simulink model "F16ASYM_Controlled_AoA"  (R2012b)
settings: Solver=ode3  SolverMode=SingleTasking  StartTime=0.0  StopTime=inf  FixedStep=T_sim  RelTol=1e-3
InitFcn:
  | load('NN_c_weights_Last_stable.mat')
values from neighbouring files (symbols this model uses):
  K_b_AoA = params(3)    [Cost_function.m]
  K_b_q = params(4)    [Cost_function.m]
  learning = 20    [Scheduling_desing.m]
  Model_used_flag = 1    [Scheduling_desing.m]
  reg_param = 0.5    [Scheduling_desing.m]
  T_sim = 0.02    [Scheduling_desing.m]
  tau_AoA = params(1)    [Cost_function.m]
  tau_q = params(2)    [Cost_function.m]
  Theta_1_roll_last = [0.00183613313267 0.00115998993235 0.0006676025148 0.00194921904952 0.00134963559861 0.00034352059664 0.000447169388141 0.00146749660935 0.00110199952389 7.77922383894e-05 0.00109492833348 0.00192687590535 ... (360 elements, 30x12)]    [NN_i_weights_LAST_STABLE.mat]
  Theta_2_roll_last = [0.000469743069697 0.000355923851088 0.00180035760697 0.00191855117771 0.00118851504447 0.0013331642065 0.0013164316578 0.000643981263341 0.00176817665434 0.000113802099363 0.000426534542462 0.00113815782354 ... (620 elements, 20x31)]    [NN_i_weights_LAST_STABLE.mat]
  Theta_3_roll_last = [9.62071520568e-05 -0.000389870886846 2.08260845013e-05 0.000140787743673 -0.000917525755397 -0.0014324207578 -0.00154701573815 -0.00131544476264 -0.00101205584381 5.06515794689e-05 -0.00111443483676 -0.00143957416141 ... (21 elements, 1x21)]    [NN_i_weights_LAST_STABLE.mat]
  V_long_lastA_w_z = [0.352826086601 -0.253633004548 -0.642535042878 0.237749930435 -0.618390629538 0.858074761295 0.268211230628 -0.448715080196 -0.0406384631192 0.401147605577 0.60598427709 0.0500551915851 ... (300 elements, 30x10)]    [NN_i_weights_LAST_STABLE.mat]
  V_long_lastAoA = [0.0774300162379 0.0911421319631 0.0352371192557 0.0542170286952 0.0651171200844 0.0177112012707 0.0982957728448 0.000259994642558 0.0194724569123 0.0466321328252 0.0556687953852 0.0252668067142 ... (300 elements, 30x10)]    [NN_i_weights_LAST_STABLE.mat]
  V_roll_last = [0.0540918675943 0.0557493347212 0.0839792276608 0.0460576391794 0.0671229058124 0.100220403067 0.0722493281881 0.0648875457457 0.00447599349201 0.0607299103823 0.0488037966361 0.0176785979393 ... (360 elements, 30x12)]    [NN_i_weights_LAST_STABLE.mat]
  V_yaw_last = [0.0965149149679 0.00833616709545 0.0365734360076 0.0523944217566 0.00790252078455 0.0700053845887 0.0345164868709 0.0111568465295 0.094060639546 0.0205483560006 0.000798047494256 0.0862769385758 ... (360 elements, 30x12)]    [NN_i_weights_LAST_STABLE.mat]
  velocity = M_eval_sche(I,J)*a    [Scheduling_desing.m]
  W_long_lastA_w_z = [-0.0522913429974 0.00385484301394 -0.00465489482472 -0.0139416219936 0.00295196421483 -0.013027768541 0.00585545058915 0.00278802233571 -0.00906272782329 -0.000396112031465 0.00405849743321 0.00509668457818 ... (31 elements, 1x31)]    [NN_i_weights_LAST_STABLE.mat]
  W_long_lastAoA = [-0.0192589013922 0.00873109909713 0.00432649597332 0.0420946902441 0.0293366820194 0.0351497798191 0.0234952374236 0.0360841187718 0.0112233388211 0.030147202199 0.0369533138617 0.00218839076415 ... (31 elements, 1x31)]    [NN_i_weights_LAST_STABLE.mat]
  W_roll_last = [-0.0006515532842 0.000535485585715 0.000550946920743 0.000806030945453 0.00045976209382 0.00065557954304 0.000945902185602 0.00070191398535 0.000635215543728 4.66501377412e-05 0.000597079583757 0.000485790566765 ... (31 elements, 1x31)]    [NN_i_weights_LAST_STABLE.mat]
  W_yaw_last = [-4.34263633305e-05 8.83823048922e-05 1.65575463724e-05 3.60293102233e-05 5.19752447623e-05 7.06399280852e-06 7.02425975821e-05 3.62680255076e-05 1.29996379937e-05 8.05072914397e-05 2.39941870661e-05 2.52427840574e-06 ... (31 elements, 1x31)]    [NN_i_weights_LAST_STABLE.mat]
undefined symbols (not defined in the file or in its folder): a1, alpha_map_eval, B, beta_map_eval, C_L_0, DiscIntNeverNeededParam, fi_flag_Simulink, G_eval, H_sq, H_sq_autotrim, k_B, m_B, M_sq, M_sq_autotrim, sigbuilder_block, Stall_curve, trim_control, trim_state, trim_throttle, V_Comp_A_w_z_last, V_Comp_last, V_roll_lastMOD, W_Comp_A_w_z_last, W_Comp_last, W_roll_lastMOD
libraries: Adaptive_FaultTolerantControl x43, dspsigops x29, F16_Actuator_Library x14, simulink x8, aerolibatmos2 x7, dsparch4 x6, simulink_extras x5, aerolibtransform2 x5, qcatlib x4, dspmtrx3 x3, dspvision x2, dspsnks4 x2
(part 6 of 11)

== system F16ASYM_Controlled_AoA/Primary Controller/P controller + adaptive Crossed NN/Lat_dir Dyn Inversion: beta_dot->r_c ==
  beta_dot_c : Inport
  All_meas : Inport  Port=2
  A_w_y : Selector  InputPortWidth=3  IndexOptions=Index vector (dialog)  Indices=2  OutputSizes=1
  Bus Selector : BusSelector  OutputSignals=signal1.AoA meas (rad),signal1.omega_b meas (rad/s),signal1.V_TAS (m/s),signal2.A_w_CG
  Divide1 : Product  Inputs=**
  Divide3 : Product  Inputs=**
  Divide4 : Product  Inputs=/*
  Divide5 : Product  Inputs=*/
  Selector : Selector  InputPortWidth=3  IndexOptions=Index vector (dialog)  Indices=1  OutputSizes=1
  Trigonometric Function : Trigonometry  Operator=cos
  Trigonometric Function3 : Trigonometry  Operator=tan
  "q_c " : Sum  Inputs=-++
  r_c : Outport
  wires:
  Selector/1 -> Divide1/2
  Trigonometric Function3/1 -> Divide1/1
  beta_dot_c/1 -> Divide5/1
  Divide5/1 -> "q_c "/1
  Trigonometric Function/1 -> Divide5/2, Divide3/1
  Bus Selector/3 -> Divide3/2  "<V_TAS (m/s)>"
  Divide4/1 -> "q_c "/3
  Bus Selector/4 -> A_w_y/1  "<A_w_CG>"
  All_meas/1 -> Bus Selector/1
  A_w_y/1 -> Divide4/2
  Divide3/1 -> Divide4/1
  Divide1/1 -> "q_c "/2
  Bus Selector/2 -> Selector/1  "<omega_b meas (rad/s)>"
  Bus Selector/1 -> Trigonometric Function3/1, Trigonometric Function/1  "<AoA meas (rad)>"
  "q_c "/1 -> r_c/1

== system F16ASYM_Controlled_AoA/Primary Controller/P controller + adaptive Crossed NN/Long Dyn Inversion: alpha_dot ->q ==
  alpha_dot_c : Inport
  All_meas : Inport  Port=2
  Completed : Subsystem
  Manual Switch : ManualSwitch
  Simplified : Subsystem
  q_c : Outport
  wires:
  Manual Switch/1 -> q_c/1
  Simplified/1(q_c) -> Manual Switch/2
  Completed/1(q_c) -> Manual Switch/1
  All_meas/1 -> Completed/2(All_meas), Simplified/2(All_meas)
  alpha_dot_c/1 -> Completed/1(alpha_dot_c), Simplified/1(alpha_dot_c)

== system F16ASYM_Controlled_AoA/Primary Controller/P controller + adaptive Crossed NN/Longitudinal Controller: AoA or A_w_z ==
  A_w_z des : Inport
  AoA des (rad) : Inport  Port=2
  Anti-windup A_w_z : Inport  Port=3
  Anti-windup AoA : Inport  Port=4
  All meas : Inport  Port=5
  Longitudinal controller in A_w_z : Subsystem  VariantObject=Controller of A_w_z
  Longitudinal controller in AoA : Subsystem  VariantObject=Controller of AoA
  A_chanel vars : Outport
  alpha_chanel vars : Outport  Port=2
  alpha_dot_c : Outport  Port=3

== system F16ASYM_Controlled_AoA/Primary Controller/P controller + adaptive Crossed NN/Sigmoid  ==
  In : Inport
  Display : Display
  Fcn1 : Fcn  Commented=on  Expr=2.0 ./ (1.0 + exp(-u(4)*u(1:3)))-1
  MATLAB Function : MATLAB Function  TreatAsAtomicUnit=on
  a : Constant  Value=a
  Out : Outport
  wires:
  a/1 -> MATLAB Function/2(a)
  In/1 -> MATLAB Function/1(u)
  MATLAB Function/1(y) -> Out/1, Display/1

== system F16ASYM_Controlled_AoA/Primary Controller/P controller + adaptive Crossed NN + AWU+Lim /Body Rates Controller ==
  p_ref : Inport
  q_ref : Inport  Port=2
  r_ref : Inport  Port=3
  All_meas : Inport  Port=4
  Bus Creator : BusCreator
  Bus Creator1 : BusCreator
  Bus Creator2 : BusCreator
  Bus Selector : BusSelector  OutputSignals=signal1.omega_b meas (rad/s)
  Display1 : Display
  Mux : Mux  Inputs=3
  Ref Model and P Controller p : Adaptive_FaultTolerantControl/Ref Model and P Controller  tau=0.1  y_i=trim_state(10)  K_f=1  K_b=7
  Ref Model and P Controller q : Adaptive_FaultTolerantControl/Ref Model and P Controller  tau=0.25  y_i=trim_state(11)  K_f=1  K_b=6
  Ref Model and P Controller r : Adaptive_FaultTolerantControl/Ref Model and P Controller  tau=0.2  y_i=trim_state(12)  K_f=1  K_b=4
  Selector : Selector  InputPortWidth=3  IndexOptions=Index vector (dialog)  Indices=1  OutputSizes=1
  Selector1 : Selector  InputPortWidth=3  IndexOptions=Index vector (dialog)  Indices=2  OutputSizes=1
  Selector2 : Selector  InputPortWidth=3  IndexOptions=Index vector (dialog)  Indices=3  OutputSizes=1
  Sum : Sum  Inputs=+-|
  Sum1 : Sum  Inputs=+-|
  Sum2 : Sum  Inputs=+-|
  q_chanel vars : Outport
  p_chanel vars : Outport  Port=2
  r_chanel vars : Outport  Port=3
  Angular acc des (rad/s^2) : Outport  Port=4
  wires:
  All_meas/1 -> Bus Selector/1
  Bus Selector/1 -> Selector/1, Selector1/1, Selector2/1  "<omega_b meas (rad/s)>"
  p_ref/1 -> Ref Model and P Controller p/1
  Selector/1 -> Ref Model and P Controller p/2
  Ref Model and P Controller p/1 -> Mux/1
  Mux/1 -> Angular acc des (rad/s^2)/1
  q_ref/1 -> Ref Model and P Controller q/1
  Selector1/1 -> Ref Model and P Controller q/2
  r_ref/1 -> Ref Model and P Controller r/1
  Ref Model and P Controller q/1 -> Mux/2
  Ref Model and P Controller r/1 -> Mux/3
  Ref Model and P Controller p/2 -> Bus Creator/1  "p_sf_dot"
  Ref Model and P Controller p/3 -> Sum/1, Bus Creator/2  "p_sf"
  Sum/1 -> Display1/1, Bus Creator/3  "p_err"
  Bus Creator/1 -> p_chanel vars/1
  Bus Creator1/1 -> q_chanel vars/1
  Bus Creator2/1 -> r_chanel vars/1
  Selector2/1 -> Ref Model and P Controller r/2
  Ref Model and P Controller p/4 -> Sum/2
  Ref Model and P Controller p/5 -> Bus Creator/4  "K_b_p"
  Ref Model and P Controller q/2 -> Bus Creator1/1  "q_sf_dot"
  Ref Model and P Controller q/3 -> Sum1/1, Bus Creator1/2  "q_sf"
  Sum1/1 -> Bus Creator1/3  "q_err"
  Ref Model and P Controller q/4 -> Sum1/2
  Ref Model and P Controller q/5 -> Bus Creator1/4  "K_b_q"
  Ref Model and P Controller r/2 -> Bus Creator2/1  "r_sf_dot"
  Ref Model and P Controller r/3 -> Sum2/1, Bus Creator2/2  "r_sf"
  Sum2/1 -> Bus Creator2/3  "r_err"
  Ref Model and P Controller r/4 -> Sum2/2
  Ref Model and P Controller r/5 -> Bus Creator2/4  "K_b_r"

== system F16ASYM_Controlled_AoA/Primary Controller/P controller + adaptive Crossed NN + AWU+Lim /Complete crossed On-line (adaptive) multi-layer NN ==
  v_ad^ prev : Inport
  All_meas : Inport  Port=2
  NN variables : Inport  Port=3
  AWU : Inport  Port=4
  Complete crossed On-line (adaptive) multi-layer NN: A_w_z : Subsystem  VariantObject=NN on A_w_z
  Complete crossed On-line (adaptive) multi-layer NN: AoA : Subsystem  VariantObject=NN on AoA
  v_ad^ : Outport

== system F16ASYM_Controlled_AoA/Primary Controller/P controller + adaptive Crossed NN + AWU+Lim /Lat_dir Dyn Inversion: beta_dot->r_c ==
  beta_dot_c : Inport
  All_meas : Inport  Port=2
  A_w_y : Selector  InputPortWidth=3  IndexOptions=Index vector (dialog)  Indices=2  OutputSizes=1
  Bus Selector : BusSelector  OutputSignals=signal1.AoA meas (rad),signal1.omega_b meas (rad/s),signal1.V_TAS (m/s),signal2.A_w_CG
  Divide1 : Product  Inputs=**
  Divide3 : Product  Inputs=**
  Divide4 : Product  Inputs=/*
  Divide5 : Product  Inputs=*/
  Selector : Selector  InputPortWidth=3  IndexOptions=Index vector (dialog)  Indices=1  OutputSizes=1
  Trigonometric Function : Trigonometry  Operator=cos
  Trigonometric Function3 : Trigonometry  Operator=tan
  "q_c " : Sum  Inputs=-++
  r_c : Outport
  wires:
  "q_c "/1 -> r_c/1
  Bus Selector/1 -> Trigonometric Function/1, Trigonometric Function3/1  "<AoA meas (rad)>"
  Bus Selector/2 -> Selector/1  "<omega_b meas (rad/s)>"
  Divide1/1 -> "q_c "/2
  Divide3/1 -> Divide4/1
  A_w_y/1 -> Divide4/2
  All_meas/1 -> Bus Selector/1
  Bus Selector/4 -> A_w_y/1  "<A_w_CG>"
  Divide4/1 -> "q_c "/3
  Bus Selector/3 -> Divide3/2  "<V_TAS (m/s)>"
  Trigonometric Function/1 -> Divide3/1, Divide5/2
  Divide5/1 -> "q_c "/1
  beta_dot_c/1 -> Divide5/1
  Trigonometric Function3/1 -> Divide1/1
  Selector/1 -> Divide1/2

== system F16ASYM_Controlled_AoA/Primary Controller/P controller + adaptive Crossed NN + AWU+Lim /Long Dyn Inversion: alpha_dot ->q ==
  alpha_dot_c : Inport
  All_meas : Inport  Port=2
  Completed : Subsystem
  Manual Switch : ManualSwitch
  Simplified : Subsystem
  q_c : Outport
  wires:
  alpha_dot_c/1 -> Simplified/1(alpha_dot_c), Completed/1(alpha_dot_c)
  All_meas/1 -> Simplified/2(All_meas), Completed/2(All_meas)
  Completed/1(q_c) -> Manual Switch/1
  Simplified/1(q_c) -> Manual Switch/2
  Manual Switch/1 -> q_c/1

== system F16ASYM_Controlled_AoA/Primary Controller/P controller + adaptive Crossed NN + AWU+Lim /Longitudinal Controller: AoA or A_w_z ==
  A_w_z des : Inport
  AoA des (rad) : Inport  Port=2
  Anti-windup A_w_z : Inport  Port=3
  Anti-windup AoA : Inport  Port=4
  All meas : Inport  Port=5
  Longitudinal controller in A_w_z : Subsystem  VariantObject=Controller of A_w_z
  Longitudinal controller in AoA : Subsystem  VariantObject=Controller of AoA
  A_chanel vars : Outport
  alpha_chanel vars : Outport  Port=2
  alpha_dot_c : Outport  Port=3

== system F16ASYM_Controlled_AoA/Primary Controller/P controller + adaptive Crossed NN + AWU+Lim /Physical limitation ==
  note: Converto to Angular accelerations
  v comm : Inport
  all meas : Inport  Port=2
  Ang Accel : MATLAB Function
  Bus Selector : BusSelector  OutputSignals=signal1.Alt meas (m),signal1.V_TAS (m/s),signal1.AoA meas (rad),signal1.SS meas (rad),signal1.omega_b meas (rad/s),signal1.Throttle_meas
  Bus Selector1 : BusSelector  OutputSignals=signal2.q (Pa),signal1.omega_b meas (rad/s)
  Demux : Demux  Outputs=3
  Display : Display
  Display1 : Display
  Display2 : Display
  Divide : Product  Inputs=**
  Divide1 : Product  Inputs=**
  Gain : Gain  Gain=-1
  Gain1 : Gain
  Mom coefficients that was reached : MATLABFcn  MATLABFcn=Moms_Coeff_estimator  OutputDimensions=3  OutputSignalType=real
  Moments : Subsystem
  Mux : Mux  Inputs=3
  Mux1 : Mux  Inputs=7
  Saturation Dynamic : simulink/Discontinuities/Saturation Dynamic  OutMin=[]  OutMax=[]  OutDataTypeStr=Inherit: Same as second input  OutDataType=fixdt(1, 16)  OutScaling=2^-10  DoSatur=off
  Sign : Signum
  Sign1 : Signum
  max deflections estimator : MATLAB Function  TreatAsAtomicUnit=on
  v limted : Outport
  wires:
  max deflections estimator/1(max_defl) -> Mux1/7
  Mux1/1 -> Mom coefficients that was reached/1
  Bus Selector/5 -> Mux1/5  "<omega_b meas (rad/s)>"
  Bus Selector/1 -> Mux1/1  "<Alt meas (m)>"
  Bus Selector/2 -> Mux1/2  "<V_TAS (m/s)>"
  Bus Selector/3 -> Mux1/3  "<AoA meas (rad)>"
  Bus Selector/4 -> Mux1/4  "<SS meas (rad)>"
  Bus Selector/6 -> Mux1/6  "<Throttle_meas>"
  Ang Accel/2(q_dot) -> Mux/2
  Ang Accel/3(r_dot) -> Mux/3
  Ang Accel/1(p_dot) -> Mux/1
  Bus Selector1/2 -> Ang Accel/4(omega_b)  "<omega_b meas (rad/s)>"
  Moments/3(N) -> Ang Accel/3(N)
  Moments/2(M) -> Ang Accel/2(M)
  Moments/1(L) -> Ang Accel/1(L)
  Bus Selector1/1 -> Moments/4(q)  "<q (Pa)>"
  Demux/3 -> Moments/3(C_N)
  Demux/2 -> Moments/2(C_M)
  Demux/1 -> Moments/1(C_L)
  Mom coefficients that was reached/1 -> Demux/1
  all meas/1 -> Bus Selector/1, Bus Selector1/1
  Mux/1 -> Gain1/1
  v comm/1 -> Saturation Dynamic/2, Display1/1, max deflections estimator/1(v_comm)
  Saturation Dynamic/1 -> Display/1, v limted/1
  Sign/1 -> Divide/1
  Gain1/1 -> Divide/2, Divide1/1, Sign1/1, Display2/1, Sign/1
  Sign1/1 -> Gain/1
  Divide/1 -> Saturation Dynamic/1
  Gain/1 -> Divide1/2
  Divide1/1 -> Saturation Dynamic/3

== system F16ASYM_Controlled_AoA/Primary Controller/P controller + adaptive Crossed NN + AWU+Lim /Sigmoid  ==
  In : Inport
  Display : Display
  Fcn1 : Fcn  Commented=on  Expr=2.0 ./ (1.0 + exp(-u(4)*u(1:3)))-1
  MATLAB Function : MATLAB Function  TreatAsAtomicUnit=on
  a : Constant  Value=a
  Out : Outport
  wires:
  MATLAB Function/1(y) -> Display/1, Out/1
  In/1 -> MATLAB Function/1(u)
  a/1 -> MATLAB Function/2(a)

== system F16ASYM_Controlled_AoA/Primary Controller/P controller + adaptive Isolated NN/Body Rates Controller ==
  p_ref : Inport
  q_ref : Inport  Port=2
  r_ref : Inport  Port=3
  All_meas : Inport  Port=4
  Bus Creator : BusCreator
  Bus Creator1 : BusCreator
  Bus Creator2 : BusCreator
  Bus Selector : BusSelector  OutputSignals=signal1.omega_b meas (rad/s)
  Display1 : Display
  Mux : Mux  Inputs=3
  Ref Model and P Controller p : Adaptive_FaultTolerantControl/Ref Model and P Controller  tau=0.1  y_i=trim_state(10)  K_f=1  K_b=7
  Ref Model and P Controller q : Adaptive_FaultTolerantControl/Ref Model and P Controller  tau=0.25  y_i=trim_state(11)  K_f=1  K_b=8
  Ref Model and P Controller r : Adaptive_FaultTolerantControl/Ref Model and P Controller  tau=0.2  y_i=trim_state(12)  K_f=1  K_b=4
  Selector : Selector  InputPortWidth=3  IndexOptions=Index vector (dialog)  Indices=1  OutputSizes=1
  Selector1 : Selector  InputPortWidth=3  IndexOptions=Index vector (dialog)  Indices=2  OutputSizes=1
  Selector2 : Selector  InputPortWidth=3  IndexOptions=Index vector (dialog)  Indices=3  OutputSizes=1
  Sum : Sum  Inputs=+-|
  Sum1 : Sum  Inputs=+-|
  Sum2 : Sum  Inputs=+-|
  q_chanel vars : Outport
  p_chanel vars : Outport  Port=2
  r_chanel vars : Outport  Port=3
  Angular acc des (rad/s^2) : Outport  Port=4
  wires:
  All_meas/1 -> Bus Selector/1
  Bus Selector/1 -> Selector/1, Selector1/1, Selector2/1  "<omega_b meas (rad/s)>"
  p_ref/1 -> Ref Model and P Controller p/1
  Selector/1 -> Ref Model and P Controller p/2
  Ref Model and P Controller p/1 -> Mux/1
  Mux/1 -> Angular acc des (rad/s^2)/1
  q_ref/1 -> Ref Model and P Controller q/1
  Selector1/1 -> Ref Model and P Controller q/2
  r_ref/1 -> Ref Model and P Controller r/1
  Ref Model and P Controller q/1 -> Mux/2
  Ref Model and P Controller r/1 -> Mux/3
  Ref Model and P Controller p/2 -> Bus Creator/1  "p_sf_dot"
  Ref Model and P Controller p/3 -> Sum/1, Bus Creator/2  "p_sf"
  Sum/1 -> Display1/1, Bus Creator/3  "p_err"
  Bus Creator/1 -> p_chanel vars/1
  Bus Creator1/1 -> q_chanel vars/1
  Bus Creator2/1 -> r_chanel vars/1
  Selector2/1 -> Ref Model and P Controller r/2
  Ref Model and P Controller p/4 -> Sum/2
  Ref Model and P Controller p/5 -> Bus Creator/4  "K_b_p"
  Ref Model and P Controller q/2 -> Bus Creator1/1  "q_sf_dot"
  Ref Model and P Controller q/3 -> Sum1/1, Bus Creator1/2  "q_sf"
  Sum1/1 -> Bus Creator1/3  "q_err"
  Ref Model and P Controller q/4 -> Sum1/2
  Ref Model and P Controller q/5 -> Bus Creator1/4  "K_b_q"
  Ref Model and P Controller r/2 -> Bus Creator2/1  "r_sf_dot"
  Ref Model and P Controller r/3 -> Sum2/1, Bus Creator2/2  "r_sf"
  Sum2/1 -> Bus Creator2/3  "r_err"
  Ref Model and P Controller r/4 -> Sum2/2
  Ref Model and P Controller r/5 -> Bus Creator2/4  "K_b_r"

== system F16ASYM_Controlled_AoA/Primary Controller/P controller + adaptive Isolated NN/Lat_dir Dyn Inversion: beta_dot->r_c ==
  beta_dot_c : Inport
  All_meas : Inport  Port=2
  A_w_y : Selector  InputPortWidth=3  IndexOptions=Index vector (dialog)  Indices=2  OutputSizes=1
  Bus Selector : BusSelector  OutputSignals=signal1.AoA meas (rad),signal1.omega_b meas (rad/s),signal1.V_TAS (m/s),signal2.A_w_CG
  Divide1 : Product  Inputs=**
  Divide3 : Product  Inputs=**
  Divide4 : Product  Inputs=/*
  Divide5 : Product  Inputs=*/
  Selector : Selector  InputPortWidth=3  IndexOptions=Index vector (dialog)  Indices=1  OutputSizes=1
  Trigonometric Function : Trigonometry  Operator=cos
  Trigonometric Function3 : Trigonometry  Operator=tan
  "q_c " : Sum  Inputs=-++
  r_c : Outport
  wires:
  "q_c "/1 -> r_c/1
  Bus Selector/1 -> Trigonometric Function/1, Trigonometric Function3/1  "<AoA meas (rad)>"
  Bus Selector/2 -> Selector/1  "<omega_b meas (rad/s)>"
  Divide1/1 -> "q_c "/2
  Divide3/1 -> Divide4/1
  A_w_y/1 -> Divide4/2
  All_meas/1 -> Bus Selector/1
  Bus Selector/4 -> A_w_y/1  "<A_w_CG>"
  Divide4/1 -> "q_c "/3
  Bus Selector/3 -> Divide3/2  "<V_TAS (m/s)>"
  Trigonometric Function/1 -> Divide3/1, Divide5/2
  Divide5/1 -> "q_c "/1
  beta_dot_c/1 -> Divide5/1
  Trigonometric Function3/1 -> Divide1/1
  Selector/1 -> Divide1/2

== system F16ASYM_Controlled_AoA/Primary Controller/P controller + adaptive Isolated NN/Long Dyn Inversion: alpha_dot ->q ==
  alpha_dot_c : Inport
  All_meas : Inport  Port=2
  Completed : Subsystem
  Manual Switch : ManualSwitch
  Simplified : Subsystem
  q_c : Outport
  wires:
  alpha_dot_c/1 -> Simplified/1(alpha_dot_c), Completed/1(alpha_dot_c)
  All_meas/1 -> Simplified/2(All_meas), Completed/2(All_meas)
  Completed/1(q_c) -> Manual Switch/1
  Simplified/1(q_c) -> Manual Switch/2
  Manual Switch/1 -> q_c/1

== system F16ASYM_Controlled_AoA/Primary Controller/P controller + adaptive Isolated NN/Longitudinal Controller: AoA or A_w_z ==
  A_w_z des : Inport
  AoA des (rad) : Inport  Port=2
  Anti-windup A_w_z : Inport  Port=3
  Anti-windup AoA : Inport  Port=4
  All meas : Inport  Port=5
  Longitudinal controller in A_w_z : Subsystem  VariantObject=Controller of A_w_z
  Longitudinal controller in AoA : Subsystem  VariantObject=Controller of AoA
  A_chanel vars : Outport
  alpha_chanel vars : Outport  Port=2
  alpha_dot_c : Outport  Port=3

== system F16ASYM_Controlled_AoA/Primary Controller/P controller + adaptive Isolated NN/On-line (adaptive) multi-layer NNs ==
  v_ad^ prev : Inport
  All_meas : Inport  Port=2
  NN variables : Inport  Port=3
  Bus Selector : BusSelector  OutputSignals=p_chanel_vars,Long chanel,beta_r_chanel
  Long Chanel : Subsystem  Variant=on  OverrideUsingVariant=Long HL NN A_w_z
  Long_learning rate : Constant  Value=30.5  SampleTime=T_sim
  Long_reg param : Constant  SampleTime=T_sim
  Mux : Mux  Inputs=3
  Roll NN : Subsystem  Variant=on  OverrideUsingVariant=Roll 2HL NN
  Roll_learning rate : Constant  Value=73  SampleTime=T_sim
  Roll_reg param : Constant  SampleTime=T_sim
  Selector : Selector  InputPortWidth=3  IndexOptions=Index vector (dialog)  Indices=1  OutputSizes=1
  Selector1 : Selector  InputPortWidth=3  IndexOptions=Index vector (dialog)  Indices=2  OutputSizes=1
  Selector2 : Selector  InputPortWidth=3  IndexOptions=Index vector (dialog)  Indices=3  OutputSizes=1
  Yaw Chanel : Subsystem  Variant=on  OverrideUsingVariant=Yaw HL NN
  Yaw_learning rate : Constant  Value=20.8  SampleTime=T_sim
  Yaw_reg param : Constant  Value=0.8  SampleTime=T_sim
  v_ad^ prev1 : InportShadow
  v_ad^ prev2 : InportShadow
  v_ad^ : Outport
  wires:
  NN variables/1 -> Bus Selector/1
  Bus Selector/1 -> Roll NN/2(p_chanel vars)  "<p_chanel_vars>"
  All_meas/1 -> Yaw Chanel/3(All_meas), Long Chanel/3(All_meas), Roll NN/3(All_meas)
  Roll NN/1(v_ad_comp) -> Mux/1
  Mux/1 -> v_ad^/1
  v_ad^ prev/1 -> Selector/1
  Selector/1 -> Roll NN/1(v_ad^ prev)
  Roll_learning rate/1 -> Roll NN/4(Roll_learning rate)
  Roll_reg param/1 -> Roll NN/5(Roll reg param)
  Selector1/1 -> Long Chanel/1(v_ad^ prev)
  Long_learning rate/1 -> Long Chanel/4(Long_learning rate)
  Long_reg param/1 -> Long Chanel/5(Long reg param)
  v_ad^ prev1/1 -> Selector1/1
  Bus Selector/2 -> Long Chanel/2(Long_chanel vars)  "<Long chanel>"
  Yaw_learning rate/1 -> Yaw Chanel/4(Yaw_learning rate)
  Yaw_reg param/1 -> Yaw Chanel/5(Yaw reg param)
  v_ad^ prev2/1 -> Selector2/1
  Selector2/1 -> Yaw Chanel/1(v_ad^ prev)
  Bus Selector/3 -> Yaw Chanel/2(Yaw_chanel vars)  "<beta_r_chanel>"
  Yaw Chanel/1(v_ad_comp) -> Mux/3
  Long Chanel/1(v_ad_comp) -> Mux/2

== system F16ASYM_Controlled_AoA/Primary Controller/P controller + adaptive Isolated NN/On-line (adaptive) multi-layer NNs SIMPL ==
  v_ad^ prev : Inport
  All_meas : Inport  Port=2
  NN variables : Inport  Port=3
  Bus Selector : BusSelector  OutputSignals=p_chanel_vars,Long chanel,beta_r_chanel
  Long Chanel : Subsystem  Variant=on  OverrideUsingVariant=Long HL NN A_w_z
  Long_learning rate : Constant  Value=19.7  SampleTime=T_sim
  Long_reg param : Constant  Value=0.9  SampleTime=T_sim
  Mux : Mux  Inputs=3
  Roll NN : Subsystem  Variant=on  OverrideUsingVariant=Roll 1HL NN
  Roll_learning rate : Constant  Value=80  SampleTime=T_sim
  Roll_reg param : Constant  Value=0.5  SampleTime=T_sim
  Selector : Selector  InputPortWidth=3  IndexOptions=Index vector (dialog)  Indices=1  OutputSizes=1
  Selector1 : Selector  InputPortWidth=3  IndexOptions=Index vector (dialog)  Indices=2  OutputSizes=1
  Selector2 : Selector  InputPortWidth=3  IndexOptions=Index vector (dialog)  Indices=3  OutputSizes=1
  Yaw Chanel : Subsystem  Variant=on  OverrideUsingVariant=Yaw HL NN
  Yaw_learning rate : Constant  Value=20.5  SampleTime=T_sim
  Yaw_reg param : Constant  SampleTime=T_sim
  v_ad^ prev1 : InportShadow
  v_ad^ prev2 : InportShadow
  v_ad^ : Outport
  wires:
  Long Chanel/1(v_ad_comp) -> Mux/2
  Yaw Chanel/1(v_ad_comp) -> Mux/3
  Bus Selector/3 -> Yaw Chanel/2(Yaw_chanel vars)  "<beta_r_chanel>"
  Selector2/1 -> Yaw Chanel/1(v_ad^ prev)
  v_ad^ prev2/1 -> Selector2/1
  Yaw_reg param/1 -> Yaw Chanel/5(Yaw reg param)
  Yaw_learning rate/1 -> Yaw Chanel/4(Yaw_learning rate)
  Bus Selector/2 -> Long Chanel/2(Long_chanel vars)  "<Long chanel>"
  v_ad^ prev1/1 -> Selector1/1
  Long_reg param/1 -> Long Chanel/5(Long reg param)
  Long_learning rate/1 -> Long Chanel/4(Long_learning rate)
  Selector1/1 -> Long Chanel/1(v_ad^ prev)
  Roll_reg param/1 -> Roll NN/5(Roll reg param)
  Roll_learning rate/1 -> Roll NN/4(Roll_learning rate)
  Selector/1 -> Roll NN/1(v_ad^ prev)
  v_ad^ prev/1 -> Selector/1
  Mux/1 -> v_ad^/1
  Roll NN/1(v_ad_comp) -> Mux/1
  All_meas/1 -> Roll NN/3(All_meas), Long Chanel/3(All_meas), Yaw Chanel/3(All_meas)
  Bus Selector/1 -> Roll NN/2(p_chanel vars)  "<p_chanel_vars>"
  NN variables/1 -> Bus Selector/1

== system F16ASYM_Controlled_AoA/Primary Controller/P controller + adaptive Isolated NN/Sigmoid  ==
  In : Inport
  Display : Display
  Fcn1 : Fcn  Commented=on  Expr=2.0 ./ (1.0 + exp(-u(4)*u(1:3)))-1
  MATLAB Function : MATLAB Function  TreatAsAtomicUnit=on
  a : Constant  Value=a
  Out : Outport
  wires:
  MATLAB Function/1(y) -> Display/1, Out/1
  In/1 -> MATLAB Function/1(u)
  a/1 -> MATLAB Function/2(a)

== system F16ASYM_Controlled_AoA/Primary Controller/PI Primary Controller/Body Rates Controller ==
  p_ref : Inport
  q_ref : Inport  Port=2
  r_ref : Inport  Port=3
  All_meas : Inport  Port=4
  All Anti-windup signals : Inport  Port=5
  Bus Creator : BusCreator  Inputs=3
  Bus Creator1 : BusCreator  Inputs=3
  Bus Creator2 : BusCreator  Inputs=3
  Bus Selector : BusSelector  OutputSignals=signal1.omega_b meas (rad/s)
  Display : Display
  Mux : Mux  Inputs=3
  Ref Model and PI Controller P : Adaptive_FaultTolerantControl/Ref Model and PI Controller  delta=0  tau=0.2  y_i=trim_state(10)  K_f=0.8  K_a=3  Con_way=pro  omega_n=4  xi=0.5  Z1=-30  K_b=10  f_i=0.2  f_c=1
  Ref Model and PI Controller q : Adaptive_FaultTolerantControl/Ref Model and PI Controller  delta=trim_state(11)  tau=0.15  y_i=0  K_f=0.8  K_a=3  Con_way=pro  omega_n=4  xi=0.5  Z1=-30  K_b=5  f_i=0.1  f_c=1
  Ref Model and PI Controller r : Adaptive_FaultTolerantControl/Ref Model and PI Controller  delta=trim_state(12)  tau=0.2  y_i=0  K_f=0.8  K_a=3  Con_way=pro  omega_n=4  xi=0.5  Z1=-30  K_b=10  f_i=0.2  f_c=1
  Selector : Selector  InputPortWidth=3  IndexOptions=Index vector (dialog)  Indices=1  OutputSizes=1
  Selector1 : Selector  InputPortWidth=3  IndexOptions=Index vector (dialog)  Indices=2  OutputSizes=1
  Selector2 : Selector  InputPortWidth=3  IndexOptions=Index vector (dialog)  Indices=3  OutputSizes=1
  Selector3 : Selector  InputPortWidth=3  IndexOptions=Index vector (dialog)  Indices=1  OutputSizes=1
  Selector4 : Selector  InputPortWidth=3  IndexOptions=Index vector (dialog)  Indices=2  OutputSizes=1
  Selector5 : Selector  InputPortWidth=3  IndexOptions=Index vector (dialog)  Indices=3  OutputSizes=1
  Sum : Sum  Inputs=|+-
  Sum1 : Sum  Inputs=|+-
  Sum2 : Sum  Inputs=|+-
  Terminator : Terminator
  Terminator1 : Terminator
  Terminator2 : Terminator
  Angular acc des (rad/s^2) : Outport
  wires:
  Bus Creator2/1 -> Terminator2/1
  Sum2/1 -> Bus Creator2/3  "r_err"
  Ref Model and PI Controller r/4 -> Sum2/2
  Ref Model and PI Controller r/3 -> Bus Creator2/2, Sum2/1  "r_sf"
  Ref Model and PI Controller r/2 -> Bus Creator2/1  "r_sf_dot"
  Bus Creator1/1 -> Terminator1/1
  Sum1/1 -> Bus Creator1/3  "q_err"
  Ref Model and PI Controller q/4 -> Sum1/2
  Ref Model and PI Controller q/3 -> Bus Creator1/2, Sum1/1  "q_sf"
  Ref Model and PI Controller q/2 -> Bus Creator1/1  "q_sf_dot"
  Bus Creator/1 -> Terminator/1
  Sum/1 -> Bus Creator/3  "p_err"
  Ref Model and PI Controller P/4 -> Sum/2
  Ref Model and PI Controller P/3 -> Bus Creator/2, Sum/1  "p_sf"
  Ref Model and PI Controller P/2 -> Bus Creator/1  "p_sf_dot"
  Selector3/1 -> Ref Model and PI Controller P/3
  Selector5/1 -> Ref Model and PI Controller r/3
  Selector4/1 -> Ref Model and PI Controller q/3, Display/1
  All Anti-windup signals/1 -> Selector3/1, Selector5/1, Selector4/1
  Ref Model and PI Controller r/1 -> Mux/3
  Ref Model and PI Controller q/1 -> Mux/2
  r_ref/1 -> Ref Model and PI Controller r/1
  Selector2/1 -> Ref Model and PI Controller r/2
  Selector1/1 -> Ref Model and PI Controller q/2
  q_ref/1 -> Ref Model and PI Controller q/1
  Mux/1 -> Angular acc des (rad/s^2)/1
  Ref Model and PI Controller P/1 -> Mux/1
  Selector/1 -> Ref Model and PI Controller P/2
  p_ref/1 -> Ref Model and PI Controller P/1
  Bus Selector/1 -> Selector/1, Selector1/1, Selector2/1  "<omega_b meas (rad/s)>"
  All_meas/1 -> Bus Selector/1

== system F16ASYM_Controlled_AoA/Primary Controller/PI Primary Controller/Lat_dir Dyn Inversion: beta_dot->r_c ==
  beta_dot_c : Inport
  All_meas : Inport  Port=2
  A_w_y : Selector  InputPortWidth=3  IndexOptions=Index vector (dialog)  Indices=2  OutputSizes=1
  Bus Selector : BusSelector  OutputSignals=signal1.AoA meas (rad),signal1.omega_b meas (rad/s),signal1.V_TAS (m/s),signal2.A_w_CG
  Divide1 : Product  Inputs=**
  Divide3 : Product  Inputs=**
  Divide4 : Product  Inputs=/*
  Divide5 : Product  Inputs=*/
  Selector : Selector  InputPortWidth=3  IndexOptions=Index vector (dialog)  Indices=1  OutputSizes=1
  Trigonometric Function : Trigonometry  Operator=cos
  Trigonometric Function3 : Trigonometry  Operator=tan
  "q_c " : Sum  Inputs=-++
  r_c : Outport
  wires:
  Selector/1 -> Divide1/2
  Trigonometric Function3/1 -> Divide1/1
  beta_dot_c/1 -> Divide5/1
  Divide5/1 -> "q_c "/1
  Trigonometric Function/1 -> Divide5/2, Divide3/1
  Bus Selector/3 -> Divide3/2  "<V_TAS (m/s)>"
  Divide4/1 -> "q_c "/3
  Bus Selector/4 -> A_w_y/1  "<A_w_CG>"
  All_meas/1 -> Bus Selector/1
  A_w_y/1 -> Divide4/2
  Divide3/1 -> Divide4/1
  Divide1/1 -> "q_c "/2
  Bus Selector/2 -> Selector/1  "<omega_b meas (rad/s)>"
  Bus Selector/1 -> Trigonometric Function3/1, Trigonometric Function/1  "<AoA meas (rad)>"
  "q_c "/1 -> r_c/1

== system F16ASYM_Controlled_AoA/Primary Controller/PI Primary Controller/Long Dyn Inversion: alpha_dot ->q ==
  alpha_dot_c : Inport
  All_meas : Inport  Port=2
  Completed : Subsystem
  Manual Switch : ManualSwitch
  Simplified : Subsystem
  q_c : Outport
  wires:
  Manual Switch/1 -> q_c/1
  Simplified/1(q_c) -> Manual Switch/2
  Completed/1(q_c) -> Manual Switch/1
  All_meas/1 -> Completed/2(All_meas), Simplified/2(All_meas)
  alpha_dot_c/1 -> Completed/1(alpha_dot_c), Simplified/1(alpha_dot_c)

== system F16ASYM_Controlled_AoA/Primary Controller/PI Primary Controller/Longitudinal Controller: AoA or A_w_z ==
  A_w_z des : Inport
  AoA des (rad) : Inport  Port=2
  Anti-windup A_w_z : Inport  Port=3
  Anti-windup AoA : Inport  Port=4
  All meas : Inport  Port=5
  Longitudinal controller in A_w_z : Subsystem  VariantObject=Controller of A_w_z
  Longitudinal controller in AoA : Subsystem  VariantObject=Controller of AoA
  alpha_dot_c : Outport

== system F16ASYM_Controlled_AoA/SI and FDI/SI and FDI: Realistic/FDI: Assumed? ==
  note: Add noise, uncertainty and delay here!!!
  note: RECONFIGURATION PARAMETERS
      |
      | 24. mass  Estimated mass
      | 25. S_current_L
      | 26. S_current_R
      | 27. S_fin_current
      | 28. x_cg
      | 29. Jy
      | 30. Jxz
      | 31. Jz
      | 32. Jx
      | 33. EFF_el_L
      | 34. EFF_el_R
      | 35. EFF_ail_L
      | 36. EFF_ail_R
      | 37. EFF_rud
      | 38. EFF_lef_L
      | 39. EFF_lef_R
      | 40. Delta_C_Lift_X
      | 41. Delta_C_Drag_X
      | 42. Delta_C_m_X
  Inexistent Reconfig bus : Inport
  All  meas : Inport  Port=2
  Bus Selector : BusSelector  OutputSignals=Reconfig signal,Blockades,Blockade now
  ONLY Effectiveness : Selector  InputPortWidth=19  IndexOptions=Index vector (dialog)  Indices=10:16  OutputSizes=1
  Terminator : Terminator
  Blockades at : Outport
  Blockades now : Outport  Port=2
  Effectiveness : Outport  Port=3
  wires:
  ONLY Effectiveness/1 -> Effectiveness/1
  Bus Selector/3 -> Blockades now/1  "<Blockade now>"
  Bus Selector/2 -> Blockades at/1  "<Blockades>"
  Bus Selector/1 -> ONLY Effectiveness/1  "<Reconfig signal>"
  Inexistent Reconfig bus/1 -> Bus Selector/1
  All  meas/1 -> Terminator/1

== system F16ASYM_Controlled_AoA/SI and FDI/SI and FDI: Realistic/SI ==
  note: Include here a logic that takes into account P so if the estimation is very bad do something
  note: Something to be done here!!!
  note: No estimation on this yet
  note: No estimation on this yet
  note: INPUTS
      | States:
      |
      | 1. Altitude
      | 2. TAS velocity
      | 3. alpha in rad
      | 4. beta in rads
      | 5. P
      | 6. Q
      | 7. R
      | 8. Throttle
      | 9. Elevator_L in deg
      | 10. Elevator_R in deg
      | 11. Aileron_L
      | 12. Aileron_R
      | 13. Rudder
      | 14. LEF_L
      | 15. LEF_R
      |
      | RECONFIGURATION PARAMETERS
      |
      | 16. mass  Estimated mass
      | 17. S_current_L
      | 18. S_current_R
      | 19. S_fin_current
      | 20. x_cg
      | 21. Jy
      | 22. Jxz
      | 23. Jz
      | 24. Jx
      | 25. EFF_el_L
      | 26. EFF_el_R
      | 27. EFF_ail_L
      | 28 EFF_ail_R
      | 29. EFF_rud
      | 30. EFF_lef_L
      | 31. EFF_lef_R
      | 32. Delta_C_Lift_X
      | 33. Delta_C_Drag_X
      | 34. Delta_C_m_X
  Control Eff : Inport
  All meas : Inport  Port=2
  Control comms : Inport  Port=3
  Add : Sum
  Band-Limited White Noise : simulink/Sources/Band-Limited White Noise  Cov=0.0000005  Ts=T_sim  seed=[23341]
  Base-line model parameters : Constant  Commented=on  Value=[9295.44,27.87/2,27.87/2,6.578,0.3,75673.6,1331.4,85552.1,12874.8]
  Bus Selector1 : BusSelector  OutputSignals=signal1.Alt meas (m),signal1.V_TAS (m/s),signal1.AoA meas (rad),signal1.SS meas (rad),signal1.omega_b meas (rad/s)
  Bus Selector2 : BusSelector  OutputSignals=signal1.omega_b meas (rad/s)
  Demux : Demux  Outputs=3
  Derivative : Derivative  CoefficientInTFapproximation=900
  Mass properties estimated : Constant  Value=[9295.44,0.3,75673.6,1331.4,85552.1,12874.8]
  Memory : Memory  X0=1*eye(3)
  Memory1 : Memory  X0=[27.87/2,27.87/2,6.578]
  Mux : Mux  Inputs=3
  Mux1 : Mux  Inputs=3
  NO-deviations from base-line model : Constant  Value=zeros(1,3)
  Scope : Scope
      settings: ShowLegends=on  YMin=1  YMax=15  SaveName=ScopeData23
  Scope1 : Scope
      settings: YMin=-2.75  YMax=3  SaveName=ScopeData24
  Surfaces UKF estimator : MATLAB Function  TreatAsAtomicUnit=on
  f(x)  Mom Coefficients due to the dynamics: Coefficients model with control inputs : MATLABFcn  Commented=on  MATLABFcn=Moms_Coeff_Reconf_estimator  OutputDimensions=3  OutputSignalType=real
  Est Mass props : Outport
  Est Surfs : Outport  Port=2
  Est Aero changes : Outport  Port=3
  wires:
  Mass properties estimated/1 -> Est Mass props/1
  All meas/1 -> Bus Selector1/1, Bus Selector2/1
  Control Eff/1 -> Surfaces UKF estimator/10(Ctrl_effectiveness)
  Control comms/1 -> Surfaces UKF estimator/9(Control_def)
  Bus Selector1/1 -> Surfaces UKF estimator/4(Alt)  "<Alt meas (m)>"
  Bus Selector1/2 -> Surfaces UKF estimator/5(TAS)  "<V_TAS (m/s)>"
  Bus Selector1/3 -> Surfaces UKF estimator/6(AoA)  "<AoA meas (rad)>"
  Bus Selector1/4 -> Surfaces UKF estimator/7(SS)  "<SS meas (rad)>"
  Bus Selector1/5 -> Surfaces UKF estimator/8(omega_b)  "<omega_b meas (rad/s)>"
  Surfaces UKF estimator/2(S_l) -> Mux/1
  Surfaces UKF estimator/3(S_r) -> Mux/2
  Surfaces UKF estimator/4(S_f) -> Mux/3
  Mux/1 -> Demux/1, Est Surfs/1, Memory1/1
  Surfaces UKF estimator/1(P_out) -> Memory/1
  NO-deviations from base-line model/1 -> Surfaces UKF estimator/11(Deltas_Aero), Est Aero changes/1
  Memory/1 -> Surfaces UKF estimator/1(P)
  Memory1/1 -> Surfaces UKF estimator/2(X_ant)
  Bus Selector2/1 -> Add/2  "<omega_b meas (rad/s)>"
  Derivative/1 -> Scope1/1, Surfaces UKF estimator/3(Meas)
  Band-Limited White Noise/1 -> Add/1
  Add/1 -> Derivative/1
  Demux/1 -> Mux1/1  "Left_wing"
  Demux/2 -> Mux1/2  "Right_wing"
  Demux/3 -> Mux1/3  "Fin"
  Mux1/1 -> Scope/1

== system F16ASYM_Controlled_AoA/Stall protection A_z and AoA/AoA and load factor map/If Action Subsystem ==
  Action Port : ActionPort
  From Multimedia File : dspvision/From Multimedia File  inputFilename=C:\Users\David\Documents\Estudios y formación academica\Cranfield\Thesis F16\Work\Solutions\7dof Development\Used Functions\Stall_warning.mp3  loop=on  numPlays=inf  outputStreams=Audio only  videoDataType=single  audioDataType=int16  inheritSampleTime=off  userDefinedSampleTime=T_sim  noAudioOutput=off  isIntensityVideo=off  fourcc=RGB  colorVideoFormat=Separate color signals  outputEOF=off  dataOrg=Column-major  audioFrameSize=1024  computeAudioFrameSize=off  outSamplingMode=Frame based
  To Audio Device : dspsnks4/To Audio Device  deviceName=Default  inheritSampleRate=on  sampleRate=44100  deviceDatatype=Determine from input data type  autoBufferSize=on  bufferSize=4096  queueDuration=1.0
  wires:
  From Multimedia File/1 -> To Audio Device/1

== system F16ASYM_Controlled_AoA/Stall protection A_z and AoA/Using AoA/Prediction ==
  V_TAS : Inport
  Add : Sum
  Derivative : Derivative  CoefficientInTFapproximation=20
  T_pred : Gain  Gain=T_pred
  V_tas pred : Outport
  wires:
  V_TAS/1 -> Add/1, Derivative/1
  Derivative/1 -> T_pred/1
  T_pred/1 -> Add/2
  Add/1 -> V_tas pred/1

== system F16ASYM_Controlled_AoA/Stall protection A_z and AoA/Using AoA/Speed stall logic ==
  stall signal : Inport
  Clock : Clock
  Constant : Constant  Value=-0.5/5  SampleTime=-1
  Constant1 : Constant  Value=0
  Discrete-Time Integrator : DiscreteIntegrator  ExternalReset=rising  InitialCondition=1  SampleTime=T_sim  LimitOutput=on  UpperSaturationLimit=1  LowerSaturationLimit=0  ICPrevOutput=DiscIntNeverNeededParam  ICPrevScaledInput=DiscIntNeverNeededParam
  pusher : Switch  Threshold=11
  timered signal : Outport
  wires:
  stall signal/1 -> Discrete-Time Integrator/2
  Constant/1 -> Discrete-Time Integrator/1
  Discrete-Time Integrator/1 -> pusher/1
  pusher/1 -> timered signal/1
  Clock/1 -> pusher/2
  Constant1/1 -> pusher/3

== system F16ASYM_Controlled_AoA/Stall protection A_z and AoA/Using AoA/play stall warning ==
  Action Port : ActionPort  InitializeStates=reset  ActionType=then
  From Multimedia File : dspvision/From Multimedia File  inputFilename=C:\Users\David\Documents\Estudios y formación academica\Cranfield\Thesis F16\Work\Solutions\7dof Development\Used Functions\Stall_warning.mp3  loop=on  numPlays=inf  outputStreams=Audio only  videoDataType=single  audioDataType=int16  inheritSampleTime=off  userDefinedSampleTime=T_sim  noAudioOutput=off  isIntensityVideo=off  fourcc=RGB  colorVideoFormat=Separate color signals  outputEOF=off  dataOrg=Column-major  audioFrameSize=1024  computeAudioFrameSize=off  outSamplingMode=Frame based
  To Audio Device : dspsnks4/To Audio Device  deviceName=Default  inheritSampleRate=on  sampleRate=44100  deviceDatatype=Determine from input data type  autoBufferSize=on  bufferSize=4096  queueDuration=1.0
  wires:
  From Multimedia File/1 -> To Audio Device/1

== system F16ASYM_Controlled_AoA/Control allocator/Control allocator: NO RECONF/Leading Edge Flap:Symetric deflection/Creating    qbar // ps ==
  alt : Inport
  V : Inport  Port=2
  ISA Atmosphere Model : aerolibatmos2/ISA Atmosphere Model  custom=off  g=9.80665  gamma=1.4  R=287.0531  L=0.0065  h_trop=11000  h_strat=20000  rho0=1.225  P0=101325  T0=288.15
  Math Function1 : Math  Operator=square  SaturateOnIntegerOverflow=on
  Product : Product  Inputs=/*  SaturateOnIntegerOverflow=on  InputSameDT=on  OutDataTypeStr=Inherit: Same as first input
  Product5 : Product  Inputs=**  SaturateOnIntegerOverflow=on  InputSameDT=on  OutDataTypeStr=Inherit: Same as first input
  Terminator : Terminator
  Terminator1 : Terminator
  r2d4 : Gain  Gain=0.5  SaturateOnIntegerOverflow=on  OutDataTypeStr=Inherit: Same as input  ParamDataTypeStr=Inherit: Same as input
  qbar / ps : Outport
  wires:
  ISA Atmosphere Model/2 -> Terminator1/1
  ISA Atmosphere Model/1 -> Terminator/1
  ISA Atmosphere Model/3 -> Product/1
  ISA Atmosphere Model/4 -> Product5/1
  Product/1 -> qbar / ps/1
  V/1 -> Math Function1/1
  Product5/1 -> Product/2  "qbar"
  r2d4/1 -> Product5/2
  Math Function1/1 -> r2d4/1
  alt/1 -> ISA Atmosphere Model/1

== matlab function F16ASYM_Controlled_AoA/Primary Controller/P controller + adaptive Crossed NN + AWU+Lim /Physical limitation/Ang Accel ==
  data: L input; p_dot output; q_dot output; r_dot output; M input; N input; omega_b input
function [p_dot,q_dot,r_dot] = Ang_accel(L,M,N,omega_b)
Jy  = 75673.6;
Jxz = 1331.4; 
Jz  = 85552.1;  
Jx  = 12874.8;
h_E = 216.9;

denom = Jx*Jz - Jxz*Jxz;

% % C1 = ((Jy - Jz)  * Jz  - (Jxz * Jxz))/ Gamma;
% % C2 = ((Jx - Jy + Jz ) * Jxz ) / Gamma;
% % C3 = Jz / Gamma;
% % C4 = Jxz / Gamma;
% % C5 = (Jz - Jx) / Jy;
% % C6 = Jxz / Jy ;
% % C7 = 1 / Jy;
% % C8 = (Jx * (Jx - Jy ) + Jxz * Jxz) / Gamma;
% % C9 = Jx / Gamma;


p_dot =  (Jz*L + Jxz*N - (Jz*(Jz-Jy)+Jxz*Jxz)*omega_b(2)*omega_b(3) + Jxz*(Jx-Jy+Jz)*omega_b(1)*omega_b(2) + Jxz*omega_b(2)*h_E)/denom;

q_dot = (M + (Jz-Jx)*omega_b(1)*omega_b(3) - Jxz*(omega_b(1)*omega_b(1)-omega_b(3)*omega_b(3)) - omega_b(3)*h_E)/Jy;


r_dot = (Jx*N + Jxz*L + (Jx*(Jx-Jy)+Jxz*Jxz)*omega_b(1)*omega_b(2) - Jxz*(Jx-Jy+Jz)*omega_b(2)*omega_b(3) +  Jx*omega_b(2)*h_E)/denom;

== matlab function F16ASYM_Controlled_AoA/Anti-windup Calculation/Anti-windup: Reconfigurable/Antiwindup calculation ==
  data: Ang_acell_comm input; AWU output; Ang_acell_achieved input; Saturations input; B input; deflections input
function AWU = AWU_calculation(Ang_acell_comm,Ang_acell_achieved,Saturations,B,deflections)
% Computing Saturation limits
sup_limit = [24,24,21,21,29,25,25]-1;
inf_limit = [-24,-24,-21,-21,-29,0,0]+1;

for i=1:7
    Saturations(i) = Saturation_smooth(abs(Saturations(i)),deflections(i),sup_limit(i),inf_limit(i));
end
Sat_B = B*Saturations;
B_max = B*ones(7,1);

AWU=zeros(3,1);

%% Method A
% % psi = 0.01; % % of the effort above the one we consider manouvreability is reduced
% % for i=1:3
% %     if i==1 && sign(deflections(3))== sign(deflections(4)) && abs(Sat_B(i))>psi*abs(B_max(i))
% %         AWU(2) = Ang_acell_comm(2) - Ang_acell_achieved(2); % we have to desaturate longitudinally not laterally
% %     elseif  i==1 && sign(deflections(3))~= sign(deflections(4)) && abs(Sat_B(i))>psi*abs(B_max(i))
% %         AWU(i) = Ang_acell_comm(i) - Ang_acell_achieved(i);
% %     elseif i~=1 && abs(Sat_B(i))>psi*abs(B_max(i))
% %         AWU(i) = Ang_acell_comm(i) - Ang_acell_achieved(i);
% %     end 
% % end

%% Method B
% % % Long
% % if Saturations(1)~=0 || Saturations(2)~=0 ||  Saturations(6)~=0 || Saturations(7)~=0 || ((Saturations(3)~=0 || Saturations(4)~=0) && sign(deflections(3))== sign(deflections(4)) ) 
% %     AWU(2) = Ang_acell_comm(2) - Ang_acell_achieved(2);
% % end
% % % Lat-dir
% % if ((Saturations(3)~=0 || Saturations(4)~=0) && sign(deflections(3)) ~= sign(deflections(4)) )  || Saturations(5)~=0 || Saturations(6)~=0 || Saturations(7)~=0
% %     AWU(1) = Ang_acell_comm(1) - Ang_acell_achieved(1);
% %     AWU(3) = Ang_acell_comm(3) - Ang_acell_achieved(3);
% % 
% % end


%% Method C
for i=1:3
        AWU(i) = (Ang_acell_comm(i) - Ang_acell_achieved(i))*Sat_B(i)/norm(B(i,:));
end

end

function Saturation_out = Saturation_smooth(Saturation,angle,sup_limit,inf_limit)

a=5;
Saturation_out  = ( 1 - 1./(1+exp(-a*(angle-inf_limit ))) + 1./(1+exp(-a*(angle-sup_limit ))) )*Saturation;


end

== matlab function F16ASYM_Controlled_AoA/P controller + adaptive Crossed NN + AWU+Lim+scheduling   in AoA/Complete crossed On-line (adaptive) multi-layer NN: AoA/Cross NN ==
  data: X_bar input size=[25,1]; v_ad_comp output; e input; K_roll input; Ks_long input; Ks_yaw input; B input; Learnign_rate input size=1; Reg_param input size=1; AWU input; W input size=[3,51]; V input size=[50,25]; v_ad output; Z_norm_unit output; T_sim parameter; W_update output; V_update output
function [v_ad_comp,v_ad,Z_norm_unit,W_update,V_update]  = Cross_NN(X_bar,e, K_roll,Ks_long,Ks_yaw,B,Learnign_rate,Reg_param,AWU,W,V,T_sim)

%% Compute prelimiary parametes
P_roll=1/K_roll;
P_long = [   1/Ks_long(1) , 1/(Ks_long(1)^2+Ks_long(1)*Ks_long(2));
     1/(Ks_long(1)^2+Ks_long(1)*Ks_long(2)) ,(Ks_long(1)^2+Ks_long(1)*Ks_long(2)+1)/(Ks_long(2)^2*Ks_long(1)+Ks_long(2)*Ks_long(1)^2) ];
P_yaw = [   1/Ks_yaw(1) , 1/(Ks_yaw(1)^2+Ks_yaw(1)*Ks_yaw(2));
     1/(Ks_yaw(1)^2+Ks_yaw(1)*Ks_yaw(2)) ,(Ks_yaw(1)^2+Ks_yaw(1)*Ks_yaw(2)+1)/(Ks_yaw(2)^2*Ks_yaw(1)+Ks_yaw(2)*Ks_yaw(1)^2) ];
 
 P = blkdiag(P_roll,P_long,P_yaw);



zeta= e'*P*B;
% Introduce Anti-windup
K_awu = 1.2;
zeta = zeta - K_awu*AWU'.*T_sim; 
% if norm(AWU)~=0
%     Learnign_rate=0;
% end
% Convergence limitation
if norm(zeta)>2/(T_sim*Learnign_rate*Reg_param)
    zeta = (zeta./norm(zeta)).*(1.8/(T_sim*Learnign_rate*Reg_param));
end
%% Feedforward
z = V*X_bar;
s=sigmoid(V*X_bar);

sigma = [1 ; s ];
% v_ad = W*sigma;

sigma_grad = (sigma.*(ones(size(sigma))-sigma));

%% Compute the gradients or adaptation laws
Gamma_w= Learnign_rate; % W learnign rate
Gamma_v= Learnign_rate; %V learning rate
lambda = Reg_param;

V_dot=zeros(size(V));
W_dot=zeros(size(W));

W_dot= -Gamma_w*(  (sigma - sigma_grad.*[1;z] )*zeta  )';
W_dot(:,2:end)= W_dot(:,2:end) - Gamma_w*lambda*norm(zeta)*(W(:,2:end));

M = W'*zeta'.*sigma_grad ;
V_dot= -Gamma_v*( M(2:end)*X_bar'  );
V_dot(:,2:end)= V_dot(:,2:end) - Gamma_v*lambda*norm(zeta).*V(:,2:end);


% % % % Other way: Based on notes of Andrew NG
% % % 
% % % delta2=W'*zeta'.*sigma_grad;
% % % 
% % % V_dot = - Gamma_v*( delta2(2:end)*X_bar');
% % % V_dot(:,2:end)= V_dot(:,2:end) - Gamma_v*lambda*norm(zeta).*V(:,2:end);
% % % 
% % % W_dot = - Gamma_w*( sigma*zeta)';
% % % W_dot(:,2:end)= W_dot(:,2:end) - Gamma_w*lambda*norm(zeta)*(W(:,2:end));



%% Adaptation
W_update = W + T_sim*W_dot;
V_update = V + T_sim*V_dot;

%% Re-compute v_ad

s=sigmoid(V_update*X_bar);

sigma = [1 ; s(:,1) ];
v_ad = W_update*sigma;

%% Compute v_ad_comp
Z = [ V,zeros(size(V,1),size(W,2));
    zeros(size(W,1),size(V,2)),W];
    
Z_norm = norm(Z,'fro');
Z_max = 2*min(size(W,1),size(W,2) )*min( size(V,1),size(V,2) );
Z_norm_unit = Z_norm;

K_r0= 0.02;
K_r1= 0;
v_r0 = -K_r0*zeta';
v_r1 = -K_r1*(Z_norm+Z_max)*zeta';

v_ad_comp = v_ad + v_r1 +v_r0;


end

== system F16ASYM_Controlled_AoA/Control allocator/Control allocator: RECONFIG/Blockades logic: Limits injetor/Block AT INFERIOR LIMIT ==
  Limit : Inport
  Blockades : Inport  Port=2
  Demux : Demux  Outputs=7
  Mux2 : Mux  Inputs=7
  Selector : Selector  InputPortWidth=7  IndexOptions=Index vector (dialog)  Indices=1  OutputSizes=1
  Selector1 : Selector  InputPortWidth=7  IndexOptions=Index vector (dialog)  Indices=2  OutputSizes=1
  Selector2 : Selector  InputPortWidth=7  IndexOptions=Index vector (dialog)  Indices=3  OutputSizes=1
  Selector3 : Selector  InputPortWidth=7  IndexOptions=Index vector (dialog)  Indices=4  OutputSizes=1
  Selector4 : Selector  InputPortWidth=7  IndexOptions=Index vector (dialog)  Indices=5  OutputSizes=1
  Selector5 : Selector  InputPortWidth=7  IndexOptions=Index vector (dialog)  Indices=6  OutputSizes=1
  Selector6 : Selector  InputPortWidth=7  IndexOptions=Index vector (dialog)  Indices=7  OutputSizes=1
  Switch{,1..6} (7 alike) : Switch  Threshold=0.5
  isNaN{,1..6} (7 alike) : RelationalOperator  Operator=isNaN  OutDataTypeStr=boolean
  Reconfig limits : Outport
  wires:
  [Blockades] -> Selector/1
  isNaN/1 -> Switch/2
  Demux/1 -> Switch/1
  Selector/1 -> Switch/3, isNaN/1
  [Blockades] -> Selector1/1
  isNaN1/1 -> Switch1/2
  Demux/2 -> Switch1/1
  Selector1/1 -> Switch1/3, isNaN1/1
  [Blockades] -> Selector2/1
  isNaN2/1 -> Switch2/2
  Demux/3 -> Switch2/1
  Selector2/1 -> Switch2/3, isNaN2/1
  [Blockades] -> Selector3/1
  isNaN3/1 -> Switch3/2
  Demux/4 -> Switch3/1
  Selector3/1 -> Switch3/3, isNaN3/1
  [Blockades] -> Selector4/1
  isNaN4/1 -> Switch4/2
  Demux/5 -> Switch4/1
  Selector4/1 -> Switch4/3, isNaN4/1
  [Blockades] -> Selector5/1
  isNaN5/1 -> Switch5/2
  Demux/6 -> Switch5/1
  Selector5/1 -> Switch5/3, isNaN5/1
  [Blockades] -> Selector6/1
  isNaN6/1 -> Switch6/2
  Demux/7 -> Switch6/1
  Selector6/1 -> Switch6/3, isNaN6/1
  Limit/1 -> Demux/1
  Mux2/1 -> Reconfig limits/1
  Blockades/1 -> [Blockades]
  Switch/1 -> Mux2/1  "Elevator_L"
  Switch1/1 -> Mux2/2
  Switch2/1 -> Mux2/3  "Aileron_L"
  Switch3/1 -> Mux2/4  "Aileron_R"
  Switch4/1 -> Mux2/5  "Rudder"
  Switch5/1 -> Mux2/6  "LEF_L"
  Switch6/1 -> Mux2/7
